simulink model "flatball_6dof_candp_wrk"  (R2021b)
settings: Solver=ode1be  StartTime=0.0  StopTime=30  FixedStep=1e-3  MaxStep=0.01  MinStep=0.01  RelTol=1e-3
values from neighbouring files (symbols this model uses):
  amb = evalin( 'base', 'amb')    [flatball_6dof_eqom.m]
  C = evalin( 'base', 'C')    [flatball_6dof_eqom.m]
  disc = evalin( 'base', 'disc')    [flatball_6dof_eqom.m]    (also in flatball_6dof_init.m = struct; flatball_init_disc_params.m = struct)
  k_launch_F_t_release = 0.60    (= 0.6)    [flatball_6dof_hucker_init.m]
  k_launch_Fx_kd = 2e-2    (= 0.02)    [flatball_6dof_hucker_init.m]
  k_launch_Fx_ki = 15    [flatball_6dof_hucker_init.m]
  k_launch_Fx_kp = 7.5    [flatball_6dof_hucker_init.m]
  k_launch_Fx_sat_hi = 150    [flatball_6dof_hucker_init.m]
  k_launch_Fx_sat_lo = -150    [flatball_6dof_hucker_init.m]
  k_launch_Fx_t_launch_begin = 0.50    (= 0.5)    [flatball_6dof_hucker_init.m]
  k_launch_Fx_t_launch_end = k_launch_F_t_release    (= 0.6)    [flatball_6dof_hucker_init.m]
  k_launch_Fy_kd = k_launch_Fx_kd    (= 0.02)    [flatball_6dof_hucker_init.m]
  k_launch_Fy_ki = k_launch_Fx_ki    (= 15)    [flatball_6dof_hucker_init.m]
  k_launch_Fy_kp = k_launch_Fx_kp    (= 7.5)    [flatball_6dof_hucker_init.m]
  k_launch_Fy_sat_hi = k_launch_Fx_sat_hi    (= 150)    [flatball_6dof_hucker_init.m]
  k_launch_Fy_sat_lo = k_launch_Fx_sat_lo    (= -150)    [flatball_6dof_hucker_init.m]
  k_launch_Fy_t_launch_begin = 0.50    (= 0.5)    [flatball_6dof_hucker_init.m]
  k_launch_Fy_t_launch_end = k_launch_F_t_release    (= 0.6)    [flatball_6dof_hucker_init.m]
  k_launch_Fz_kd = 2.5    [flatball_6dof_hucker_init.m]
  k_launch_Fz_ki = 50    [flatball_6dof_hucker_init.m]
  k_launch_Fz_kp = 20    [flatball_6dof_hucker_init.m]
  k_launch_Fz_sat_hi = 25    [flatball_6dof_hucker_init.m]
  k_launch_Fz_sat_lo = -25    [flatball_6dof_hucker_init.m]
  k_launch_Fz_t_launch_begin = 0.10    (= 0.1)    [flatball_6dof_hucker_init.m]
  k_launch_Fz_t_launch_end = k_launch_F_t_release    (= 0.6)    [flatball_6dof_hucker_init.m]
  k_launch_M_t_release = 0.60    (= 0.6)    [flatball_6dof_hucker_init.m]
  k_launch_Mx_kd = 0.125    [flatball_6dof_hucker_init.m]
  k_launch_Mx_ki = 1.125    [flatball_6dof_hucker_init.m]
  k_launch_Mx_kp = 3.5    [flatball_6dof_hucker_init.m]
  k_launch_Mx_sat_hi = 2.5    [flatball_6dof_hucker_init.m]
  k_launch_Mx_sat_lo = -2.5    [flatball_6dof_hucker_init.m]
  k_launch_Mx_t_launch_begin = 0.30    (= 0.3)    [flatball_6dof_hucker_init.m]
  k_launch_Mx_t_launch_end = k_launch_M_t_release    (= 0.6)    [flatball_6dof_hucker_init.m]
  k_launch_My_kd = 0.1125    [flatball_6dof_hucker_init.m]
  k_launch_My_ki = 5.5    [flatball_6dof_hucker_init.m]
  k_launch_My_kp = 4.25    [flatball_6dof_hucker_init.m]
  k_launch_My_sat_hi = 2.5    [flatball_6dof_hucker_init.m]
  k_launch_My_sat_lo = -2.5    [flatball_6dof_hucker_init.m]
  k_launch_My_t_launch_begin = 0.40    (= 0.4)    [flatball_6dof_hucker_init.m]
  k_launch_My_t_launch_end = k_launch_M_t_release    (= 0.6)    [flatball_6dof_hucker_init.m]
  k_launch_Mz_kd = 1e-8    (= 1e-08)    [flatball_6dof_hucker_init.m]
  k_launch_Mz_ki = 0.2575    [flatball_6dof_hucker_init.m]
  k_launch_Mz_kp = 0.25    [flatball_6dof_hucker_init.m]
  k_launch_Mz_sat_hi = 7.5    [flatball_6dof_hucker_init.m]
  k_launch_Mz_sat_lo = -7.5    [flatball_6dof_hucker_init.m]
  k_launch_Mz_t_launch_begin = 0.20    (= 0.2)    [flatball_6dof_hucker_init.m]
  k_launch_Mz_t_launch_end = k_launch_M_t_release    (= 0.6)    [flatball_6dof_hucker_init.m]
  XL_desired = [0 0 -45*C.IN2M, 5*C.DEG2RAD 5*C.DEG2RAD 0, 15 -3 0, 0 0 500*C.RPM2RADSEC]    [flatball_6dof_wrk.m]
undefined symbols (not defined in the file or in its folder): CandP, er, flatball, flatball_6dof_plnt_lib, huck, hucker_lib
libraries: slpidlib x6, simulink x5
(part 1 of 2)
settings Model: Creator=misc.protolabs@gmail.com  LastModifiedBy=schae
settings SolverCC: InitialStep=0.01  NumberNewtonIterations=10
settings DataIOCC: SaveFormat=StructureWithTime  SaveOutput=off  DSMLogging=off  SaveTime=off  ReturnWorkspaceOutputsName=simout
settings DebuggingCC: InheritedTsInSrcMsg=none

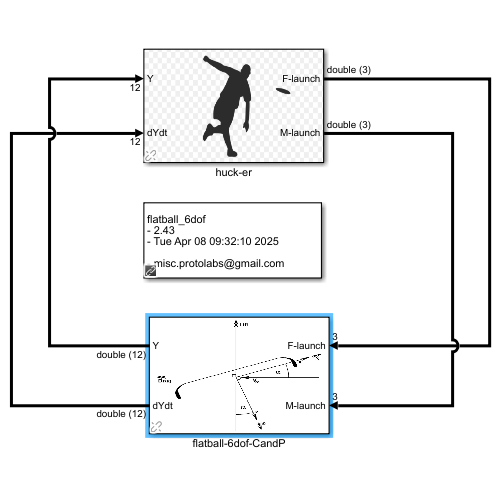
[thumbnail: Simulink's stored preview of the top-level diagram]
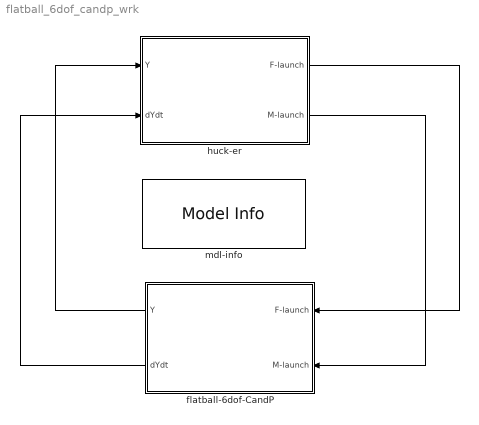
== system flatball_6dof_candp_wrk ==
  flatball-6dof-CandP : Subsystem  AncestorBlock=flatball_6dof_plnt_lib/flatball-6dof-CandP
      mask Display: image('C:\.local\desktop\flatball-dev-main-misc.protolabs\media\img\screenshots\flatball-6dof.png'); % Use "Edit Image" on toolstrip to change.
  huck-er : Subsystem  AncestorBlock=hucker_lib/huck-er
      mask Display: image('C:\.local\desktop\flatball-dev-main-misc.protolabs\media\img\screenshots\hucker.png'); % Use "Edit Image" on toolstrip to change.
  mdl-info : simulink/Model-Wide Utilities/Model Info  Frame=on  DisplayStringWithTags=|  HorizontalTextAlignment=Left  LeftAlignmentValue=0.02
      | flatball_6dof
      | - %<ModelVersion>
      | - %<LastModificationDate>
      | 
      | - %<Creator>
  wires:
  flatball-6dof-CandP/2(dYdt) -> huck-er/2(dYdt)
  flatball-6dof-CandP/1(Y) -> huck-er/1(Y)
  huck-er/1(F-launch) -> flatball-6dof-CandP/1(F-launch)
  huck-er/2(M-launch) -> flatball-6dof-CandP/2(M-launch)

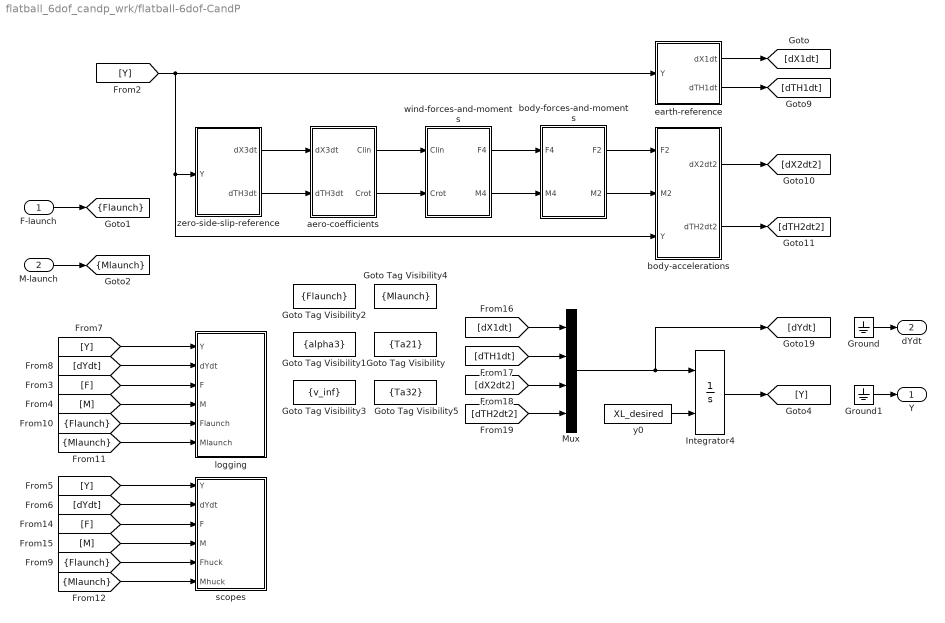
== system flatball_6dof_candp_wrk/flatball-6dof-CandP ==
  F-launch : Inport
  M-launch : Inport  Port=2
  Goto Tag Visibility : GotoTagVisibility  GotoTag=Ta21
  Goto Tag Visibility1 : GotoTagVisibility  GotoTag=alpha3
  Goto Tag Visibility2 : GotoTagVisibility  GotoTag=Flaunch
  Goto Tag Visibility3 : GotoTagVisibility  GotoTag=v_inf
  Goto Tag Visibility4 : GotoTagVisibility  GotoTag=Mlaunch
  Goto Tag Visibility5 : GotoTagVisibility  GotoTag=Ta32
  Ground : Ground
  Ground1 : Ground
  Integrator4 : Integrator  InitialConditionSource=external
  Mux : Mux
  aero-coefficients : Subsystem
  body-accelerations : Subsystem
  body-forces-and-moments : Subsystem
  earth-reference : Subsystem
  logging : Subsystem
  scopes : Subsystem
  wind-forces-and-moments : Subsystem
  y0 : Constant  Value=XL_desired
  zero-side-slip-reference : Subsystem
  Y : Outport
  dYdt : Outport  Port=2
  tag scope: Flaunch=scoped, Mlaunch=scoped
  wires:
  Ground1/1 -> Y/1
  M-launch/1 -> [Mlaunch]
  Ground/1 -> dYdt/1
  wind-forces-and-moments/2(M4) -> body-forces-and-moments/2(M4)
  body-forces-and-moments/2(M2) -> body-accelerations/2(M2)
  wind-forces-and-moments/1(F4) -> body-forces-and-moments/1(F4)
  Mux/1 -> Integrator4/1, [dYdt]
  [dX1dt] -> Mux/1
  aero-coefficients/1(Clin) -> wind-forces-and-moments/1(Clin)
  body-accelerations/1(dX2dt2) -> [dX2dt2]
  [dX2dt2] -> Mux/3
  aero-coefficients/2(Crot) -> wind-forces-and-moments/2(Crot)
  [dTH1dt] -> Mux/2
  body-forces-and-moments/1(F2) -> body-accelerations/1(F2)
  zero-side-slip-reference/2(dTH3dt) -> aero-coefficients/2(dTH3dt)
  earth-reference/1(dX1dt) -> [dX1dt]
  earth-reference/2(dTH1dt) -> [dTH1dt]
  body-accelerations/2(dTH2dt2) -> [dTH2dt2]
  [dTH2dt2] -> Mux/4
  F-launch/1 -> [Flaunch]
  Integrator4/1 -> [Y]
  zero-side-slip-reference/1(dX3dt) -> aero-coefficients/1(dX3dt)
  [Y] -> earth-reference/1(Y), body-accelerations/3(Y), zero-side-slip-reference/1(Y)
  y0/1 -> Integrator4/2
  [M] -> scopes/4(M)
  [Flaunch] -> scopes/5(Fhuck)
  [Y] -> logging/1(Y)
  [F] -> scopes/3(F)
  [Mlaunch] -> scopes/6(Mhuck)
  [M] -> logging/4(M)
  [Y] -> scopes/1(Y)
  [dYdt] -> scopes/2(dYdt)
  [Flaunch] -> logging/5(Flaunch)
  [F] -> logging/3(F)
  [Mlaunch] -> logging/6(Mlaunch)
  [dYdt] -> logging/2(dYdt)

== system flatball_6dof_candp_wrk/huck-er ==
  Y : Inport
  dYdt : Inport  Port=2
  Flaunch-ctrl : Subsystem
  Mlaunch-ctrl : Subsystem
  F-launch : Outport
  M-launch : Outport  Port=2
  wires:
  Flaunch-ctrl/1(Flaunch) -> F-launch/1
  dYdt/1 -> Flaunch-ctrl/2(dYdt), Mlaunch-ctrl/2(dYdt)
  Y/1 -> Mlaunch-ctrl/1(Y), Flaunch-ctrl/1(Y)
  Mlaunch-ctrl/1(Mlaunch) -> M-launch/1

== system flatball_6dof_candp_wrk/flatball-6dof-CandP/aero-coefficients ==
  dX3dt : Inport
  dTH3dt : Inport  Port=2
  Mux1 : Mux  Inputs=3
  Mux2 : Mux  Inputs=3
  Subsystem : Subsystem
  Subsystem1 : Subsystem
  Subsystem2 : Subsystem
  Subsystem3 : Subsystem
  Subsystem4 : Subsystem
  Subsystem5 : Subsystem
  alpha3 : Subsystem
  Clin : Outport
  Crot : Outport  Port=2
  wires:
  dX3dt/1 -> alpha3/1(dX3dt)
  Mux2/1 -> Clin/1
  dTH3dt/1 -> Subsystem3/1(dTH3dt), Subsystem2/1(dTH3dt), Subsystem4/1(dTH3dt), Subsystem5/1(dTH3dt)
  Mux1/1 -> Crot/1
  alpha3/1(alpha3) -> [alpha3]
  [alpha3] -> Subsystem/1(alpha3), Subsystem2/2(alpha3), Subsystem1/1(alpha3)
  Subsystem5/1(Cside) -> Mux2/2  "Cside"
  Subsystem/1(Cdrag) -> Mux2/1  "Cdrag"
  Subsystem1/1(Clift) -> Mux2/3  "Clift"
  Subsystem2/1(CM) -> Mux1/2  "CM"
  [v_inf] -> Subsystem5/2(v_inf), Subsystem3/2(v_inf), Subsystem2/3(v_inf), Subsystem4/2(v_inf)
  Subsystem3/1(CL) -> Mux1/1  "CL"
  Subsystem4/1(CN) -> Mux1/3  "CN"

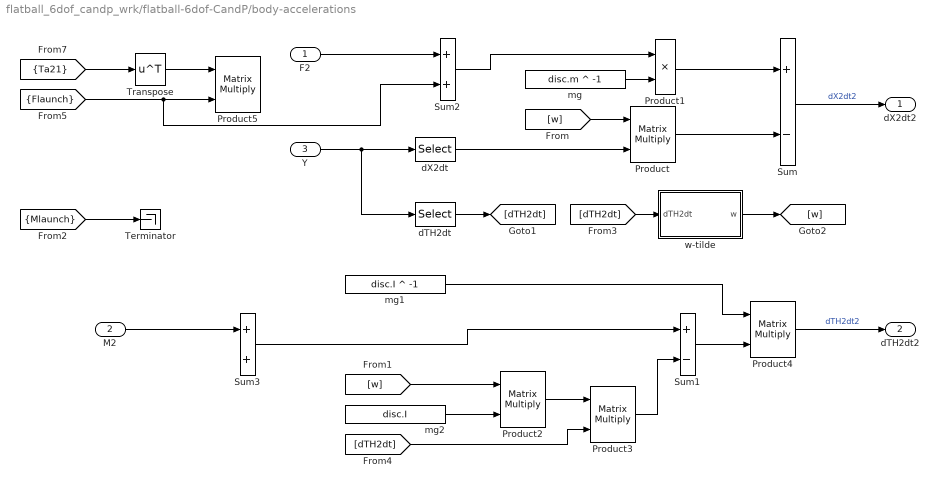
== system flatball_6dof_candp_wrk/flatball-6dof-CandP/body-accelerations ==
  F2 : Inport
  M2 : Inport  Port=2
  Y : Inport  Port=3
  Product{,2..5} (5 alike) : Product  Multiplication=Matrix(*)
  Product1 : Product  Inputs=**
  Sum : Sum  Inputs=+-
  Sum1 : Sum  Inputs=+-
  Sum2 : Sum
  Sum3 : Sum
  Terminator : Terminator
  Transpose : Math  Operator=transpose  SaturateOnIntegerOverflow=on
  dTH2dt : Selector  InputPortWidth=12  IndexOptions=Index vector (dialog)  Indices=[10 11 12]  OutputSizes=1
  dX2dt : Selector  InputPortWidth=12  IndexOptions=Index vector (dialog)  Indices=[7 8 9]  OutputSizes=1
  mg : Constant  Value=disc.m ^ -1
  mg1 : Constant  Value=disc.I ^ -1
  mg2 : Constant  Value=disc.I
  w-tilde : MATLAB Function  TreatAsAtomicUnit=on
  dX2dt2 : Outport
  dTH2dt2 : Outport  Port=2
  wires:
  Y/1 -> dTH2dt/1, dX2dt/1
  Sum/1 -> dX2dt2/1  "dX2dt2"
  Product4/1 -> dTH2dt2/1  "dTH2dt2"
  dX2dt/1 -> Product/2
  F2/1 -> Sum2/1
  mg/1 -> Product1/2
  Product1/1 -> Sum/1
  Product/1 -> Sum/2
  w-tilde/1(w) -> [w]
  [w] -> Product/1
  mg2/1 -> Product2/2
  Product2/1 -> Product3/1
  dTH2dt/1 -> [dTH2dt]
  [dTH2dt] -> w-tilde/1(dTH2dt)
  [dTH2dt] -> Product3/2
  mg1/1 -> Product4/1
  [w] -> Product2/1
  Product3/1 -> Sum1/2
  Sum1/1 -> Product4/2
  [Ta21] -> Transpose/1
  [Flaunch] -> Sum2/2, Product5/2
  Sum2/1 -> Product1/1
  Transpose/1 -> Product5/1
  [Mlaunch] -> Terminator/1
  M2/1 -> Sum3/1
  Sum3/1 -> Sum1/1

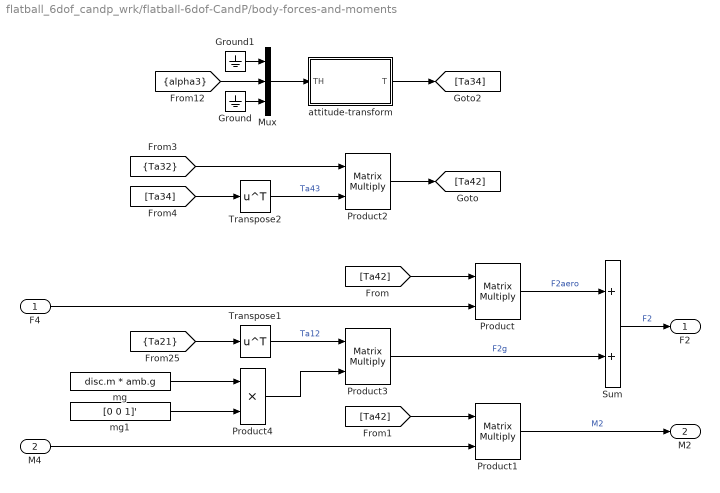
== system flatball_6dof_candp_wrk/flatball-6dof-CandP/body-forces-and-moments ==
  F4 : Inport
  M4 : Inport  Port=2
  Ground : Ground
  Ground1 : Ground
  Mux : Mux  Inputs=3
  Product{,1..3} (4 alike) : Product  Multiplication=Matrix(*)
  Product4 : Product
  Sum : Sum  Inputs=2
  Transpose1 : Math  Operator=transpose  SaturateOnIntegerOverflow=on
  Transpose2 : Math  Operator=transpose  SaturateOnIntegerOverflow=on
  attitude-transform : MATLAB Function  TreatAsAtomicUnit=on
  mg : Constant  Value=disc.m * amb.g
  mg1 : Constant  Value=[0 0 1]'
  F2 : Outport
  M2 : Outport  Port=2
  wires:
  [alpha3] -> Mux/2
  F4/1 -> Product/2
  Product/1 -> Sum/1  "F2aero"
  [Ta21] -> Transpose1/1
  Product1/1 -> M2/1  "M2"
  Ground1/1 -> Mux/1
  Mux/1 -> attitude-transform/1(TH)
  Ground/1 -> Mux/3
  attitude-transform/1(T) -> [Ta34]
  [Ta32] -> Product2/1
  [Ta34] -> Transpose2/1
  Product2/1 -> [Ta42]
  [Ta42] -> Product/1
  [Ta42] -> Product1/1
  Sum/1 -> F2/1  "F2"
  Product3/1 -> Sum/2  "F2g"
  Product4/1 -> Product3/2
  Transpose2/1 -> Product2/2  "Ta43"
  mg/1 -> Product4/1
  mg1/1 -> Product4/2
  Transpose1/1 -> Product3/1  "Ta12"
  M4/1 -> Product1/2

== system flatball_6dof_candp_wrk/flatball-6dof-CandP/earth-reference ==
  Y : Inport
  Product : Product  Multiplication=Matrix(*)
  Product1 : Product  Multiplication=Matrix(*)
  TH1 : Selector  InputPortWidth=12  IndexOptions=Index vector (dialog)  Indices=[4 5 6]  OutputSizes=1
  Terminator : Terminator
  X1 : Selector  InputPortWidth=12  IndexOptions=Index vector (dialog)  Indices=[1 2 3]  OutputSizes=1
  attitude-transform : MATLAB Function  TreatAsAtomicUnit=on
  dTH2dt : Selector  InputPortWidth=12  IndexOptions=Index vector (dialog)  Indices=[10 11 12]  OutputSizes=1
  dX2dt : Selector  InputPortWidth=12  IndexOptions=Index vector (dialog)  Indices=[7 8 9]  OutputSizes=1
  rate-transform : MATLAB Function  TreatAsAtomicUnit=on
  v_inf : Subsystem
  dX1dt : Outport
  dTH1dt : Outport  Port=2
  tag scope: Ta21=scoped
  wires:
  Y/1 -> X1/1, dTH2dt/1, dX2dt/1, TH1/1
  dX2dt/1 -> v_inf/1(dX2dt), Product/2
  TH1/1 -> rate-transform/1(TH), attitude-transform/1(TH)  "TH1"
  Product/1 -> dX1dt/1  "X1dot"
  Product1/1 -> dTH1dt/1  "TH1dot"
  X1/1 -> Terminator/1  "X1"
  attitude-transform/1(T) -> [Ta21]
  rate-transform/1(T) -> [Tr21]
  [Ta21] -> Product/1
  [Tr21] -> Product1/1
  dTH2dt/1 -> Product1/2

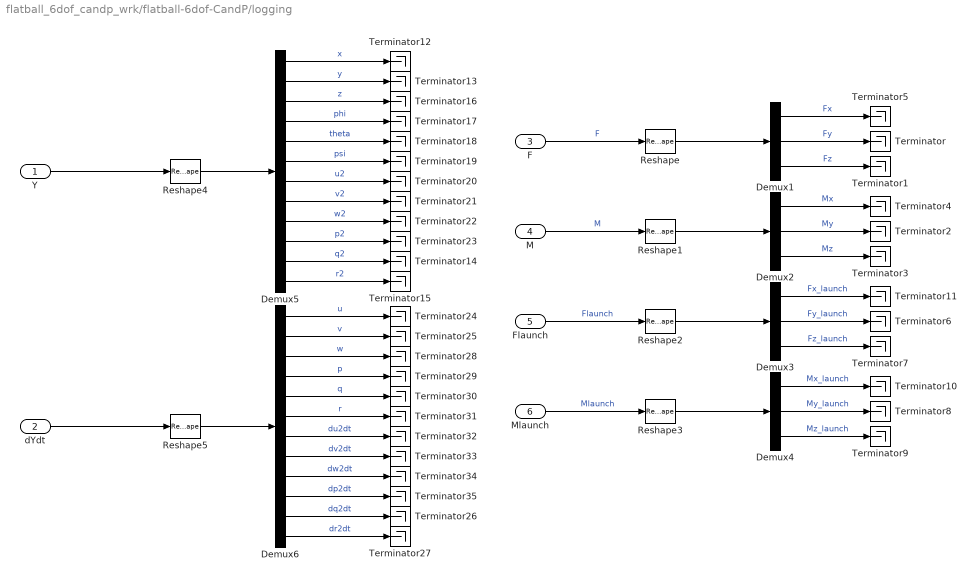
== system flatball_6dof_candp_wrk/flatball-6dof-CandP/logging ==
  Y : Inport
  dYdt : Inport  Port=2
  F : Inport  Port=3
  M : Inport  Port=4
  Flaunch : Inport  Port=5
  Mlaunch : Inport  Port=6
  Demux{1..4} (4 alike) : Demux  Outputs=3
  Demux5 : Demux  Outputs=[1 1 1 1 1 1 1 1 1 1 1 1]
  Demux6 : Demux  Outputs=[1 1 1 1 1 1 1 1 1 1 1 1]
  Reshape{,1..5} (6 alike) : Reshape
  Terminator{,1..35} (36 alike) : Terminator
  wires:
  Demux6/3 -> Terminator28/1  "w"
  Demux6/1 -> Terminator24/1  "u"
  Demux6/8 -> Terminator33/1  "dv2dt"
  Demux6/9 -> Terminator34/1  "dw2dt"
  Reshape5/1 -> Demux6/1
  Demux6/2 -> Terminator25/1  "v"
  Demux6/12 -> Terminator27/1  "dr2dt"
  Demux6/10 -> Terminator35/1  "dp2dt"
  Demux6/7 -> Terminator32/1  "du2dt"
  Demux6/5 -> Terminator30/1  "q"
  Demux6/6 -> Terminator31/1  "r"
  Demux6/11 -> Terminator26/1  "dq2dt"
  Demux6/4 -> Terminator29/1  "p"
  dYdt/1 -> Reshape5/1
  Y/1 -> Reshape4/1
  Demux5/4 -> Terminator17/1  "phi"
  Demux5/11 -> Terminator14/1  "q2"
  Demux5/6 -> Terminator19/1  "psi"
  Demux5/5 -> Terminator18/1  "theta"
  Demux5/7 -> Terminator20/1  "u2"
  Demux5/10 -> Terminator23/1  "p2"
  Demux5/12 -> Terminator15/1  "r2"
  Demux5/2 -> Terminator13/1  "y"
  Reshape4/1 -> Demux5/1
  Demux5/9 -> Terminator22/1  "w2"
  Demux5/8 -> Terminator21/1  "v2"
  Demux5/1 -> Terminator12/1  "x"
  Demux5/3 -> Terminator16/1  "z"
  Mlaunch/1 -> Reshape3/1  "Mlaunch"
  F/1 -> Reshape/1  "F"
  Demux3/2 -> Terminator6/1  "Fy_launch"
  Demux3/1 -> Terminator11/1  "Fx_launch"
  Flaunch/1 -> Reshape2/1  "Flaunch"
  Reshape3/1 -> Demux4/1
  Demux4/3 -> Terminator9/1  "Mz_launch"
  Demux4/1 -> Terminator10/1  "Mx_launch"
  Reshape/1 -> Demux1/1
  Demux1/1 -> Terminator5/1  "Fx"
  Demux4/2 -> Terminator8/1  "My_launch"
  M/1 -> Reshape1/1  "M"
  Demux3/3 -> Terminator7/1  "Fz_launch"
  Demux2/2 -> Terminator2/1  "My"
  Demux1/2 -> Terminator/1  "Fy"
  Demux1/3 -> Terminator1/1  "Fz"
  Reshape2/1 -> Demux3/1
  Demux2/1 -> Terminator4/1  "Mx"
  Demux2/3 -> Terminator3/1  "Mz"
  Reshape1/1 -> Demux2/1

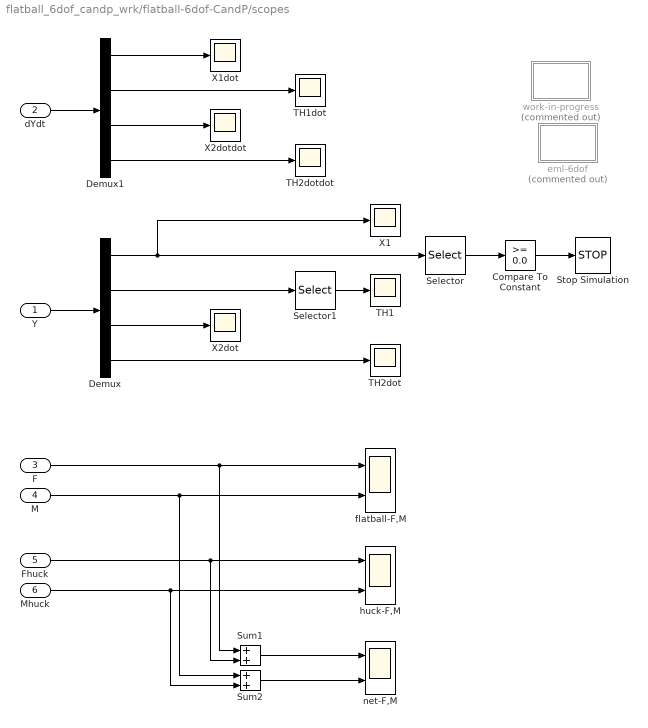
== system flatball_6dof_candp_wrk/flatball-6dof-CandP/scopes ==
  Y : Inport
  dYdt : Inport  Port=2
  F : Inport  Port=3
  M : Inport  Port=4
  Fhuck : Inport  Port=5
  Mhuck : Inport  Port=6
  Compare To Constant : simulink/Logic and Bit Operations/Compare To Constant  relop=>=  const=0.0  OutDataTypeStr=boolean
  Demux : Demux  Outputs=[3 3 3 3]
  Demux1 : Demux  Outputs=[3 3 3 3]
  Selector : Selector  InputPortWidth=3  IndexOptions=Index vector (dialog)  Indices=[3]  OutputSizes=1
  Selector1 : Selector  InputPortWidth=3  IndexOptions=Index vector (dialog)  Indices=[1 2]  OutputSizes=1
  Stop Simulation : Stop
  Sum1 : Sum
  Sum2 : Sum
  TH1 : Scope
  TH1dot : Scope
  TH2dot : Scope
  TH2dotdot : Scope
  X1 : Scope
  X1dot : Scope
  X2dot : Scope
  X2dotdot : Scope
  eml-6dof : Subsystem  Commented=on
  flatball-F,M : Scope  NumInputPorts=2
  huck-F,M : Scope  NumInputPorts=2
  net-F,M : Scope  NumInputPorts=2
  work-in-progress : Subsystem  Commented=on
  wires:
  Demux/1 -> Selector/1, X1/1
  Demux1/3 -> X2dotdot/1
  Y/1 -> Demux/1
  Compare To Constant/1 -> Stop Simulation/1
  Demux1/4 -> TH2dotdot/1
  Demux/3 -> X2dot/1
  Demux1/1 -> X1dot/1
  Selector1/1 -> TH1/1
  Demux/2 -> Selector1/1
  Demux1/2 -> TH1dot/1
  Selector/1 -> Compare To Constant/1
  dYdt/1 -> Demux1/1
  Demux/4 -> TH2dot/1
  M/1 -> flatball-F,M/2, Sum2/1
  F/1 -> flatball-F,M/1, Sum1/1
  Fhuck/1 -> huck-F,M/1, Sum1/2
  Sum1/1 -> net-F,M/1
  Mhuck/1 -> huck-F,M/2, Sum2/2
  Sum2/1 -> net-F,M/2

== system flatball_6dof_candp_wrk/flatball-6dof-CandP/wind-forces-and-moments ==
  Clin : Inport
  Crot : Inport  Port=2
  Demux : Demux  Outputs=3
  Demux1 : Demux  Outputs=3
  Gain{,1..3} (4 alike) : Gain  Gain=-1
  Gain4 : Gain  Gain=0
  Mux : Mux  Inputs=3
  Product : Product
  Product1 : Product
  Subsystem : Subsystem
  Terminator : Terminator
  Terminator1 : Terminator
  Terminator2 : Terminator
  F4 : Outport
  M4 : Outport  Port=2
  wires:
  Product/1 -> [F4], F4/1  "F4"
  Product1/1 -> M4/1  "M4"
  Demux/2 -> Terminator1/1
  Demux/1 -> Gain/1
  Demux/3 -> Gain1/1
  [F4] -> Demux/1
  Gain1/1 -> Terminator2/1  "lift"
  Gain/1 -> Terminator/1  "drag"
  Demux1/3 -> Gain3/1
  Clin/1 -> Demux1/1
  Demux1/2 -> Gain4/1
  Demux1/1 -> Gain2/1
  Gain3/1 -> Mux/3
  Gain4/1 -> Mux/2
  Gain2/1 -> Mux/1
  Mux/1 -> Product/1
  Subsystem/1(qS) -> Product/2
  Subsystem/2(qSc) -> Product1/1
  Crot/1 -> Product1/2
  [v_inf] -> Subsystem/1(v_inf)

== system flatball_6dof_candp_wrk/flatball-6dof-CandP/zero-side-slip-reference ==
  Y : Inport
  Ground : Ground
  Ground1 : Ground
  Mux : Mux  Inputs=3
  Product : Product  Multiplication=Matrix(*)
  Product1 : Product  Multiplication=Matrix(*)
  Transpose : Math  Operator=transpose  SaturateOnIntegerOverflow=on
  attitude-transform : MATLAB Function  TreatAsAtomicUnit=on
  beta2 : Subsystem
  dTH2dt : Selector  InputPortWidth=12  IndexOptions=Index vector (dialog)  Indices=[10 11 12]  OutputSizes=1
  dX2dt : Selector  InputPortWidth=12  IndexOptions=Index vector (dialog)  Indices=[7 8 9]  OutputSizes=1
  dX3dt : Outport
  dTH3dt : Outport  Port=2
  tag scope: Ta32=scoped
  wires:
  Y/1 -> dX2dt/1, dTH2dt/1
  Product1/1 -> dTH3dt/1  "dTH3dt"
  Product/1 -> dX3dt/1  "dX3dt"
  dX2dt/1 -> beta2/1(dX2dt), Product/2  "dX2dt"
  dTH2dt/1 -> Product1/2  "dTH2dt"
  beta2/1(beta2) -> Mux/3
  Mux/1 -> attitude-transform/1(TH)
  Ground/1 -> Mux/2
  Ground1/1 -> Mux/1
  attitude-transform/1(T) -> [Ta32]
  [Ta23] -> Product1/1, Product/1
  [Ta32] -> Transpose/1
  Transpose/1 -> [Ta23]  "Ta23"

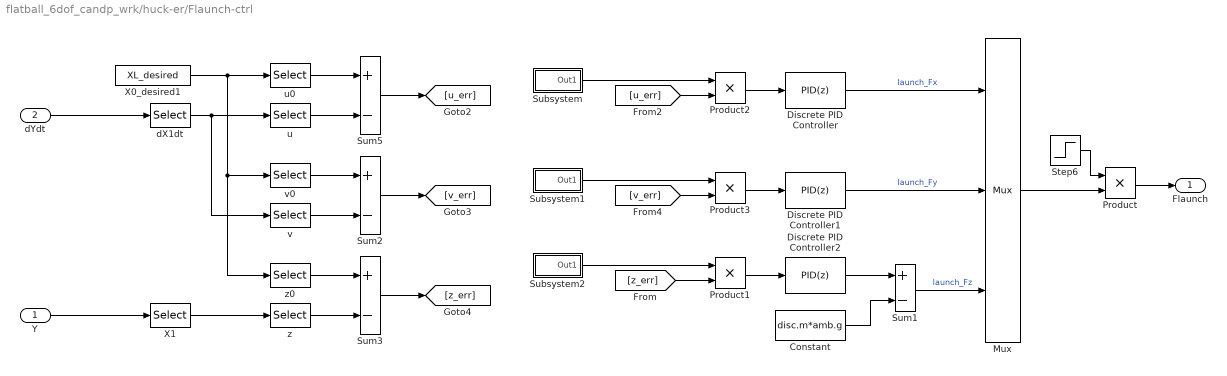
== system flatball_6dof_candp_wrk/huck-er/Flaunch-ctrl ==
  Y : Inport
  dYdt : Inport  Port=2
  Constant : Constant  Value=disc.m*amb.g
  Discrete PID Controller : slpidlib/PID Controller  Controller=PID  Form=Parallel  TimeDomain=Discrete-time  UseExternalTs=off  SampleTime=-1  IntegratorMethod=Forward Euler  FilterMethod=Forward Euler  ControllerParametersSource=internal  P=k_launch_Fx_kp  I=k_launch_Fx_ki  D=k_launch_Fx_kd  UseFilter=on  N=100  TunerSelectOption=Transfer Function Based (PID Tuner App)  InitialConditionSource=internal  InitialConditionForIntegrator=0  InitialConditionForFilter=0  DifferentiatorICPrevScaledInput=0  ExternalReset=none  TrackingMode=off  Kt=1  LimitOutput=on  SatLimitsSource=internal  UpperSaturationLimit=k_launch_Fx_sat_hi  LowerSaturationLimit=k_launch_Fx_sat_lo  LinearizeAsGain=off  AntiWindupMode=clamping  Kb=1  POutMin=[]  POutMax=[]  IOutMin=[]  IOutMax=[]  DOutMin=[]  DOutMax=[]  NOutMin=[]  NOutMax=[]  SumOutMin=[]  SumOutMax=[]  SaturationOutMin=[]  SaturationOutMax=[]  PParamMin=[]  PParamMax=[]  IParamMin=[]  IParamMax=[]  DParamMin=[]  DParamMax=[]  NParamMin=[]  NParamMax=[]  KbParamMin=[]  KbParamMax=[]  KtParamMin=[]  KtParamMax=[]  KbOutMin=[]  KbOutMax=[]  KtOutMin=[]  KtOutMax=[]  IntegratorOutMin=[]  IntegratorOutMax=[]  FilterOutMin=[]  FilterOutMax=[]  SumI1OutMin=[]  SumI1OutMax=[]  SumI2OutMin=[]  SumI2OutMax=[]  SumI3OutMin=[]  SumI3OutMax=[]  SumI4OutMin=[]  SumI4OutMax=[]  SumDOutMin=[]  SumDOutMax=[]  DifferentiatorOutMin=[]  DifferentiatorOutMax=[]  FilterDiffOutCoefMin=[]  FilterDiffOutCoefMax=[]  ReciprocalOutMin=[]  ReciprocalOutMax=[]  SumDenOutMin=[]  SumDenOutMax=[]  SumNumOutMin=[]  SumNumOutMax=[]  DivideOutMin=[]  DivideOutMax=[]  UdiffTsProdOutMin=[]  UdiffTsProdOutMax=[]  NTsProdOutMin=[]  NTsProdOutMax=[]  UintegralTsProdOutMin=[]  UintegralTsProdOutMax=[]  UngainTsProdOutMin=[]  UngainTsProdOutMax=[]  IntegratorContinuousStateAttributes=''  IntegratorStateMustResolveToSignalObject=off  IntegratorRTWStateStorageClass=Auto  FilterContinuousStateAttributes=''  FilterStateMustResolveToSignalObject=off  FilterRTWStateStorageClass=Auto  ParallelPVariant=InternalParameters  IdealPVariant=Disabled  IVariant=InternalParameters  DVariant=InternalParameters  IntegratorVariant=Discrete  SatVariant=Enabled  AWVariant=DiscClampingParallel  PCopyVariant=Disabled  TRVariant=Disabled  FdbkBlocksVariant=Forward  IdealPFdbkVariant=Disabled  SatFdbkVariant=Disabled  DerivativeFilterVariant=ForwardEulerFilter  NVariant=InternalParameters  NCopyVariant=Disabled  FilterICVariant=InternalICsFilter  IntegratorICVariant=InternalICs  ExternalResetVariant=Disabled  TRSumVariant=Passthrough  SumFdbkVariant=Disabled  SumVariant=Sum_PID  TsampFilterVariant=InternalTs  TsampNgainVariant=Passthrough  TsampIntegralVariant=Passthrough  ExternalSaturationOutDataTypeStr=Inherit: Same as second input
  Discrete PID Controller1 : slpidlib/PID Controller  Controller=PID  Form=Parallel  TimeDomain=Discrete-time  UseExternalTs=off  SampleTime=-1  IntegratorMethod=Forward Euler  FilterMethod=Forward Euler  ControllerParametersSource=internal  P=k_launch_Fy_kp  I=k_launch_Fy_ki  D=k_launch_Fy_kd  UseFilter=on  N=100  TunerSelectOption=Transfer Function Based (PID Tuner App)  InitialConditionSource=internal  InitialConditionForIntegrator=0  InitialConditionForFilter=0  DifferentiatorICPrevScaledInput=0  ExternalReset=none  TrackingMode=off  Kt=1  LimitOutput=on  SatLimitsSource=internal  UpperSaturationLimit=k_launch_Fy_sat_hi  LowerSaturationLimit=k_launch_Fy_sat_lo  LinearizeAsGain=off  AntiWindupMode=clamping  Kb=1  POutMin=[]  POutMax=[]  IOutMin=[]  IOutMax=[]  DOutMin=[]  DOutMax=[]  NOutMin=[]  NOutMax=[]  SumOutMin=[]  SumOutMax=[]  SaturationOutMin=[]  SaturationOutMax=[]  PParamMin=[]  PParamMax=[]  IParamMin=[]  IParamMax=[]  DParamMin=[]  DParamMax=[]  NParamMin=[]  NParamMax=[]  KbParamMin=[]  KbParamMax=[]  KtParamMin=[]  KtParamMax=[]  KbOutMin=[]  KbOutMax=[]  KtOutMin=[]  KtOutMax=[]  IntegratorOutMin=[]  IntegratorOutMax=[]  FilterOutMin=[]  FilterOutMax=[]  SumI1OutMin=[]  SumI1OutMax=[]  SumI2OutMin=[]  SumI2OutMax=[]  SumI3OutMin=[]  SumI3OutMax=[]  SumI4OutMin=[]  SumI4OutMax=[]  SumDOutMin=[]  SumDOutMax=[]  DifferentiatorOutMin=[]  DifferentiatorOutMax=[]  FilterDiffOutCoefMin=[]  FilterDiffOutCoefMax=[]  ReciprocalOutMin=[]  ReciprocalOutMax=[]  SumDenOutMin=[]  SumDenOutMax=[]  SumNumOutMin=[]  SumNumOutMax=[]  DivideOutMin=[]  DivideOutMax=[]  UdiffTsProdOutMin=[]  UdiffTsProdOutMax=[]  NTsProdOutMin=[]  NTsProdOutMax=[]  UintegralTsProdOutMin=[]  UintegralTsProdOutMax=[]  UngainTsProdOutMin=[]  UngainTsProdOutMax=[]  IntegratorContinuousStateAttributes=''  IntegratorStateMustResolveToSignalObject=off  IntegratorRTWStateStorageClass=Auto  FilterContinuousStateAttributes=''  FilterStateMustResolveToSignalObject=off  FilterRTWStateStorageClass=Auto  ParallelPVariant=InternalParameters  IdealPVariant=Disabled  IVariant=InternalParameters  DVariant=InternalParameters  IntegratorVariant=Discrete  SatVariant=Enabled  AWVariant=DiscClampingParallel  PCopyVariant=Disabled  TRVariant=Disabled  FdbkBlocksVariant=Forward  IdealPFdbkVariant=Disabled  SatFdbkVariant=Disabled  DerivativeFilterVariant=ForwardEulerFilter  NVariant=InternalParameters  NCopyVariant=Disabled  FilterICVariant=InternalICsFilter  IntegratorICVariant=InternalICs  ExternalResetVariant=Disabled  TRSumVariant=Passthrough  SumFdbkVariant=Disabled  SumVariant=Sum_PID  TsampFilterVariant=InternalTs  TsampNgainVariant=Passthrough  TsampIntegralVariant=Passthrough  ExternalSaturationOutDataTypeStr=Inherit: Same as second input
  Discrete PID Controller2 : slpidlib/PID Controller  Controller=PID  Form=Parallel  TimeDomain=Discrete-time  UseExternalTs=off  SampleTime=-1  IntegratorMethod=Forward Euler  FilterMethod=Forward Euler  ControllerParametersSource=internal  P=k_launch_Fz_kp  I=k_launch_Fz_ki  D=k_launch_Fz_kd  UseFilter=on  N=100  TunerSelectOption=Transfer Function Based (PID Tuner App)  InitialConditionSource=internal  InitialConditionForIntegrator=0  InitialConditionForFilter=0  DifferentiatorICPrevScaledInput=0  ExternalReset=none  TrackingMode=off  Kt=1  LimitOutput=on  SatLimitsSource=internal  UpperSaturationLimit=k_launch_Fz_sat_hi  LowerSaturationLimit=k_launch_Fz_sat_lo  LinearizeAsGain=off  AntiWindupMode=clamping  Kb=1  POutMin=[]  POutMax=[]  IOutMin=[]  IOutMax=[]  DOutMin=[]  DOutMax=[]  NOutMin=[]  NOutMax=[]  SumOutMin=[]  SumOutMax=[]  SaturationOutMin=[]  SaturationOutMax=[]  PParamMin=[]  PParamMax=[]  IParamMin=[]  IParamMax=[]  DParamMin=[]  DParamMax=[]  NParamMin=[]  NParamMax=[]  KbParamMin=[]  KbParamMax=[]  KtParamMin=[]  KtParamMax=[]  KbOutMin=[]  KbOutMax=[]  KtOutMin=[]  KtOutMax=[]  IntegratorOutMin=[]  IntegratorOutMax=[]  FilterOutMin=[]  FilterOutMax=[]  SumI1OutMin=[]  SumI1OutMax=[]  SumI2OutMin=[]  SumI2OutMax=[]  SumI3OutMin=[]  SumI3OutMax=[]  SumI4OutMin=[]  SumI4OutMax=[]  SumDOutMin=[]  SumDOutMax=[]  DifferentiatorOutMin=[]  DifferentiatorOutMax=[]  FilterDiffOutCoefMin=[]  FilterDiffOutCoefMax=[]  ReciprocalOutMin=[]  ReciprocalOutMax=[]  SumDenOutMin=[]  SumDenOutMax=[]  SumNumOutMin=[]  SumNumOutMax=[]  DivideOutMin=[]  DivideOutMax=[]  UdiffTsProdOutMin=[]  UdiffTsProdOutMax=[]  NTsProdOutMin=[]  NTsProdOutMax=[]  UintegralTsProdOutMin=[]  UintegralTsProdOutMax=[]  UngainTsProdOutMin=[]  UngainTsProdOutMax=[]  IntegratorContinuousStateAttributes=''  IntegratorStateMustResolveToSignalObject=off  IntegratorRTWStateStorageClass=Auto  FilterContinuousStateAttributes=''  FilterStateMustResolveToSignalObject=off  FilterRTWStateStorageClass=Auto  ParallelPVariant=InternalParameters  IdealPVariant=Disabled  IVariant=InternalParameters  DVariant=InternalParameters  IntegratorVariant=Discrete  SatVariant=Enabled  AWVariant=DiscClampingParallel  PCopyVariant=Disabled  TRVariant=Disabled  FdbkBlocksVariant=Forward  IdealPFdbkVariant=Disabled  SatFdbkVariant=Disabled  DerivativeFilterVariant=ForwardEulerFilter  NVariant=InternalParameters  NCopyVariant=Disabled  FilterICVariant=InternalICsFilter  IntegratorICVariant=InternalICs  ExternalResetVariant=Disabled  TRSumVariant=Passthrough  SumFdbkVariant=Disabled  SumVariant=Sum_PID  TsampFilterVariant=InternalTs  TsampNgainVariant=Passthrough  TsampIntegralVariant=Passthrough  ExternalSaturationOutDataTypeStr=Inherit: Same as second input
  Mux : Mux  Inputs=3
  Product{,1..3} (4 alike) : Product
  Step6 : Step  Time=k_launch_F_t_release  Before=1  After=0
  Subsystem : Subsystem
  Subsystem1 : Subsystem
  Subsystem2 : Subsystem
  Sum{1..3,5} (4 alike) : Sum  Inputs=+-
  X0_desired1 : Constant  Value=XL_desired
  X1 : Selector  InputPortWidth=12  IndexOptions=Index vector (dialog)  Indices=[1 2 3]  OutputSizes=1
  dX1dt : Selector  InputPortWidth=12  IndexOptions=Index vector (dialog)  Indices=[1 2 3]  OutputSizes=1
  u : Selector  InputPortWidth=3  IndexOptions=Index vector (dialog)  Indices=[1]  OutputSizes=1
  u0 : Selector  InputPortWidth=12  IndexOptions=Index vector (dialog)  Indices=[7]  OutputSizes=1
  v : Selector  InputPortWidth=3  IndexOptions=Index vector (dialog)  Indices=[2]  OutputSizes=1
  v0 : Selector  InputPortWidth=12  IndexOptions=Index vector (dialog)  Indices=[8]  OutputSizes=1
  z : Selector  InputPortWidth=3  IndexOptions=Index vector (dialog)  Indices=[3]  OutputSizes=1
  z0 : Selector  InputPortWidth=12  IndexOptions=Index vector (dialog)  Indices=[3]  OutputSizes=1
  Flaunch : Outport
  wires:
  Discrete PID Controller/1 -> Mux/1  "launch_Fx"
  Discrete PID Controller1/1 -> Mux/2  "launch_Fy"
  Sum1/1 -> Mux/3  "launch_Fz"
  Step6/1 -> Product/1
  Product/1 -> Flaunch/1
  Discrete PID Controller2/1 -> Sum1/1
  Constant/1 -> Sum1/2
  Sum5/1 -> [u_err]
  dYdt/1 -> dX1dt/1
  dX1dt/1 -> v/1, u/1
  u/1 -> Sum5/2
  X0_desired1/1 -> u0/1, z0/1, v0/1
  u0/1 -> Sum5/1
  [u_err] -> Product2/2
  Y/1 -> X1/1
  Mux/1 -> Product/2
  Sum2/1 -> [v_err]
  [v_err] -> Product3/2
  v0/1 -> Sum2/1
  v/1 -> Sum2/2
  X1/1 -> z/1
  z/1 -> Sum3/2
  z0/1 -> Sum3/1
  Sum3/1 -> [z_err]
  [z_err] -> Product1/2
  Subsystem2/1(Out1) -> Product1/1
  Product2/1 -> Discrete PID Controller/1
  Product3/1 -> Discrete PID Controller1/1
  Product1/1 -> Discrete PID Controller2/1
  Subsystem1/1(Out1) -> Product3/1
  Subsystem/1(Out1) -> Product2/1

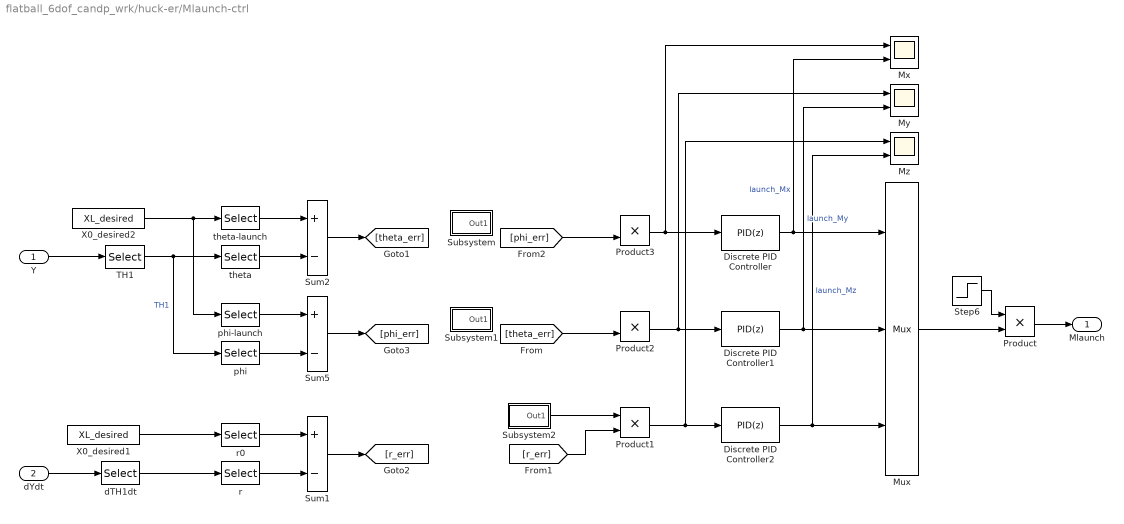
== system flatball_6dof_candp_wrk/huck-er/Mlaunch-ctrl ==
  Y : Inport
  dYdt : Inport  Port=2
  Discrete PID Controller : slpidlib/PID Controller  Controller=PID  Form=Parallel  TimeDomain=Discrete-time  UseExternalTs=off  SampleTime=-1  IntegratorMethod=Forward Euler  FilterMethod=Forward Euler  ControllerParametersSource=internal  P=k_launch_Mx_kp  I=k_launch_Mx_ki  D=k_launch_Mx_kd  UseFilter=on  N=100  TunerSelectOption=Transfer Function Based (PID Tuner App)  InitialConditionSource=internal  InitialConditionForIntegrator=0  InitialConditionForFilter=0  DifferentiatorICPrevScaledInput=0  ExternalReset=none  TrackingMode=off  Kt=1  LimitOutput=on  SatLimitsSource=internal  UpperSaturationLimit=k_launch_Mx_sat_hi  LowerSaturationLimit=k_launch_Mx_sat_lo  LinearizeAsGain=off  AntiWindupMode=clamping  Kb=1  POutMin=[]  POutMax=[]  IOutMin=[]  IOutMax=[]  DOutMin=[]  DOutMax=[]  NOutMin=[]  NOutMax=[]  SumOutMin=[]  SumOutMax=[]  SaturationOutMin=[]  SaturationOutMax=[]  PParamMin=[]  PParamMax=[]  IParamMin=[]  IParamMax=[]  DParamMin=[]  DParamMax=[]  NParamMin=[]  NParamMax=[]  KbParamMin=[]  KbParamMax=[]  KtParamMin=[]  KtParamMax=[]  KbOutMin=[]  KbOutMax=[]  KtOutMin=[]  KtOutMax=[]  IntegratorOutMin=[]  IntegratorOutMax=[]  FilterOutMin=[]  FilterOutMax=[]  SumI1OutMin=[]  SumI1OutMax=[]  SumI2OutMin=[]  SumI2OutMax=[]  SumI3OutMin=[]  SumI3OutMax=[]  SumI4OutMin=[]  SumI4OutMax=[]  SumDOutMin=[]  SumDOutMax=[]  DifferentiatorOutMin=[]  DifferentiatorOutMax=[]  FilterDiffOutCoefMin=[]  FilterDiffOutCoefMax=[]  ReciprocalOutMin=[]  ReciprocalOutMax=[]  SumDenOutMin=[]  SumDenOutMax=[]  SumNumOutMin=[]  SumNumOutMax=[]  DivideOutMin=[]  DivideOutMax=[]  UdiffTsProdOutMin=[]  UdiffTsProdOutMax=[]  NTsProdOutMin=[]  NTsProdOutMax=[]  UintegralTsProdOutMin=[]  UintegralTsProdOutMax=[]  UngainTsProdOutMin=[]  UngainTsProdOutMax=[]  IntegratorContinuousStateAttributes=''  IntegratorStateMustResolveToSignalObject=off  IntegratorRTWStateStorageClass=Auto  FilterContinuousStateAttributes=''  FilterStateMustResolveToSignalObject=off  FilterRTWStateStorageClass=Auto  ParallelPVariant=InternalParameters  IdealPVariant=Disabled  IVariant=InternalParameters  DVariant=InternalParameters  IntegratorVariant=Discrete  SatVariant=Enabled  AWVariant=DiscClampingParallel  PCopyVariant=Disabled  TRVariant=Disabled  FdbkBlocksVariant=Forward  IdealPFdbkVariant=Disabled  SatFdbkVariant=Disabled  DerivativeFilterVariant=ForwardEulerFilter  NVariant=InternalParameters  NCopyVariant=Disabled  FilterICVariant=InternalICsFilter  IntegratorICVariant=InternalICs  ExternalResetVariant=Disabled  TRSumVariant=Passthrough  SumFdbkVariant=Disabled  SumVariant=Sum_PID  TsampFilterVariant=InternalTs  TsampNgainVariant=Passthrough  TsampIntegralVariant=Passthrough  ExternalSaturationOutDataTypeStr=Inherit: Same as second input
  Discrete PID Controller1 : slpidlib/PID Controller  Controller=PID  Form=Parallel  TimeDomain=Discrete-time  UseExternalTs=off  SampleTime=-1  IntegratorMethod=Forward Euler  FilterMethod=Forward Euler  ControllerParametersSource=internal  P=k_launch_My_kp  I=k_launch_My_ki  D=k_launch_My_kd  UseFilter=on  N=100  TunerSelectOption=Transfer Function Based (PID Tuner App)  InitialConditionSource=internal  InitialConditionForIntegrator=0  InitialConditionForFilter=0  DifferentiatorICPrevScaledInput=0  ExternalReset=none  TrackingMode=off  Kt=1  LimitOutput=on  SatLimitsSource=internal  UpperSaturationLimit=k_launch_My_sat_hi  LowerSaturationLimit=k_launch_My_sat_lo  LinearizeAsGain=off  AntiWindupMode=clamping  Kb=1  POutMin=[]  POutMax=[]  IOutMin=[]  IOutMax=[]  DOutMin=[]  DOutMax=[]  NOutMin=[]  NOutMax=[]  SumOutMin=[]  SumOutMax=[]  SaturationOutMin=[]  SaturationOutMax=[]  PParamMin=[]  PParamMax=[]  IParamMin=[]  IParamMax=[]  DParamMin=[]  DParamMax=[]  NParamMin=[]  NParamMax=[]  KbParamMin=[]  KbParamMax=[]  KtParamMin=[]  KtParamMax=[]  KbOutMin=[]  KbOutMax=[]  KtOutMin=[]  KtOutMax=[]  IntegratorOutMin=[]  IntegratorOutMax=[]  FilterOutMin=[]  FilterOutMax=[]  SumI1OutMin=[]  SumI1OutMax=[]  SumI2OutMin=[]  SumI2OutMax=[]  SumI3OutMin=[]  SumI3OutMax=[]  SumI4OutMin=[]  SumI4OutMax=[]  SumDOutMin=[]  SumDOutMax=[]  DifferentiatorOutMin=[]  DifferentiatorOutMax=[]  FilterDiffOutCoefMin=[]  FilterDiffOutCoefMax=[]  ReciprocalOutMin=[]  ReciprocalOutMax=[]  SumDenOutMin=[]  SumDenOutMax=[]  SumNumOutMin=[]  SumNumOutMax=[]  DivideOutMin=[]  DivideOutMax=[]  UdiffTsProdOutMin=[]  UdiffTsProdOutMax=[]  NTsProdOutMin=[]  NTsProdOutMax=[]  UintegralTsProdOutMin=[]  UintegralTsProdOutMax=[]  UngainTsProdOutMin=[]  UngainTsProdOutMax=[]  IntegratorContinuousStateAttributes=''  IntegratorStateMustResolveToSignalObject=off  IntegratorRTWStateStorageClass=Auto  FilterContinuousStateAttributes=''  FilterStateMustResolveToSignalObject=off  FilterRTWStateStorageClass=Auto  ParallelPVariant=InternalParameters  IdealPVariant=Disabled  IVariant=InternalParameters  DVariant=InternalParameters  IntegratorVariant=Discrete  SatVariant=Enabled  AWVariant=DiscClampingParallel  PCopyVariant=Disabled  TRVariant=Disabled  FdbkBlocksVariant=Forward  IdealPFdbkVariant=Disabled  SatFdbkVariant=Disabled  DerivativeFilterVariant=ForwardEulerFilter  NVariant=InternalParameters  NCopyVariant=Disabled  FilterICVariant=InternalICsFilter  IntegratorICVariant=InternalICs  ExternalResetVariant=Disabled  TRSumVariant=Passthrough  SumFdbkVariant=Disabled  SumVariant=Sum_PID  TsampFilterVariant=InternalTs  TsampNgainVariant=Passthrough  TsampIntegralVariant=Passthrough  ExternalSaturationOutDataTypeStr=Inherit: Same as second input
  Discrete PID Controller2 : slpidlib/PID Controller  Controller=PID  Form=Parallel  TimeDomain=Discrete-time  UseExternalTs=off  SampleTime=-1  IntegratorMethod=Forward Euler  FilterMethod=Forward Euler  ControllerParametersSource=internal  P=k_launch_Mz_kp  I=k_launch_Mz_ki  D=k_launch_Mz_kd  UseFilter=on  N=100  TunerSelectOption=Transfer Function Based (PID Tuner App)  InitialConditionSource=internal  InitialConditionForIntegrator=0  InitialConditionForFilter=0  DifferentiatorICPrevScaledInput=0  ExternalReset=none  TrackingMode=off  Kt=1  LimitOutput=on  SatLimitsSource=internal  UpperSaturationLimit=k_launch_Mz_sat_hi  LowerSaturationLimit=k_launch_Mz_sat_lo  LinearizeAsGain=off  AntiWindupMode=none  Kb=1  POutMin=[]  POutMax=[]  IOutMin=[]  IOutMax=[]  DOutMin=[]  DOutMax=[]  NOutMin=[]  NOutMax=[]  SumOutMin=[]  SumOutMax=[]  SaturationOutMin=[]  SaturationOutMax=[]  PParamMin=[]  PParamMax=[]  IParamMin=[]  IParamMax=[]  DParamMin=[]  DParamMax=[]  NParamMin=[]  NParamMax=[]  KbParamMin=[]  KbParamMax=[]  KtParamMin=[]  KtParamMax=[]  KbOutMin=[]  KbOutMax=[]  KtOutMin=[]  KtOutMax=[]  IntegratorOutMin=[]  IntegratorOutMax=[]  FilterOutMin=[]  FilterOutMax=[]  SumI1OutMin=[]  SumI1OutMax=[]  SumI2OutMin=[]  SumI2OutMax=[]  SumI3OutMin=[]  SumI3OutMax=[]  SumI4OutMin=[]  SumI4OutMax=[]  SumDOutMin=[]  SumDOutMax=[]  DifferentiatorOutMin=[]  DifferentiatorOutMax=[]  FilterDiffOutCoefMin=[]  FilterDiffOutCoefMax=[]  ReciprocalOutMin=[]  ReciprocalOutMax=[]  SumDenOutMin=[]  SumDenOutMax=[]  SumNumOutMin=[]  SumNumOutMax=[]  DivideOutMin=[]  DivideOutMax=[]  UdiffTsProdOutMin=[]  UdiffTsProdOutMax=[]  NTsProdOutMin=[]  NTsProdOutMax=[]  UintegralTsProdOutMin=[]  UintegralTsProdOutMax=[]  UngainTsProdOutMin=[]  UngainTsProdOutMax=[]  IntegratorContinuousStateAttributes=''  IntegratorStateMustResolveToSignalObject=off  IntegratorRTWStateStorageClass=Auto  FilterContinuousStateAttributes=''  FilterStateMustResolveToSignalObject=off  FilterRTWStateStorageClass=Auto  ParallelPVariant=InternalParameters  IdealPVariant=Disabled  IVariant=InternalParameters  DVariant=InternalParameters  IntegratorVariant=Discrete  SatVariant=Enabled  AWVariant=Passthrough  PCopyVariant=Disabled  TRVariant=Disabled  FdbkBlocksVariant=Forward  IdealPFdbkVariant=Disabled  SatFdbkVariant=Disabled  DerivativeFilterVariant=ForwardEulerFilter  NVariant=InternalParameters  NCopyVariant=Disabled  FilterICVariant=InternalICsFilter  IntegratorICVariant=InternalICs  ExternalResetVariant=Disabled  TRSumVariant=Passthrough  SumFdbkVariant=Disabled  SumVariant=Sum_PID  TsampFilterVariant=InternalTs  TsampNgainVariant=Passthrough  TsampIntegralVariant=Passthrough  ExternalSaturationOutDataTypeStr=Inherit: Same as second input
  Mux : Mux  Inputs=3
  Mx : Scope  NumInputPorts=2
  My : Scope  NumInputPorts=2
  Mz : Scope  NumInputPorts=2
  Product{,1..3} (4 alike) : Product
  Step6 : Step  Time=k_launch_M_t_release  Before=1  After=0
  Subsystem : Subsystem
  Subsystem1 : Subsystem
  Subsystem2 : Subsystem
  Sum1 : Sum  Inputs=+-
  Sum2 : Sum  Inputs=+-
  Sum5 : Sum  Inputs=+-
  TH1 : Selector  InputPortWidth=12  IndexOptions=Index vector (dialog)  Indices=[4 5 6]  OutputSizes=1
  X0_desired1 : Constant  Value=XL_desired
  X0_desired2 : Constant  Value=XL_desired
  dTH1dt : Selector  InputPortWidth=12  IndexOptions=Index vector (dialog)  Indices=[4 5 6]  OutputSizes=1
  phi : Selector  InputPortWidth=3  IndexOptions=Index vector (dialog)  Indices=[1]  OutputSizes=1
  phi-launch : Selector  InputPortWidth=12  IndexOptions=Index vector (dialog)  Indices=[4]  OutputSizes=1
  r : Selector  InputPortWidth=3  IndexOptions=Index vector (dialog)  Indices=[3]  OutputSizes=1
  r0 : Selector  InputPortWidth=12  IndexOptions=Index vector (dialog)  Indices=[12]  OutputSizes=1
  theta : Selector  InputPortWidth=3  IndexOptions=Index vector (dialog)  Indices=[2]  OutputSizes=1
  "theta-launch " : Selector  InputPortWidth=12  IndexOptions=Index vector (dialog)  Indices=[5]  OutputSizes=1
  Mlaunch : Outport
  wires:
  Discrete PID Controller/1 -> Mux/1, Mx/2  "launch_Mx"
  Discrete PID Controller2/1 -> Mux/3, Mz/2  "launch_Mz"
  Mux/1 -> Product/2
  Step6/1 -> Product/1
  Product/1 -> Mlaunch/1
  Discrete PID Controller1/1 -> Mux/2, My/2  "launch_My"
  Product1/1 -> Discrete PID Controller2/1, Mz/1
  Product2/1 -> Discrete PID Controller1/1, My/1
  Product3/1 -> Discrete PID Controller/1, Mx/1
  Y/1 -> TH1/1
  TH1/1 -> phi/1, theta/1  "TH1"
  Subsystem2/1(Out1) -> Product1/1
  r0/1 -> Sum1/1
  dTH1dt/1 -> r/1
  r/1 -> Sum1/2
  X0_desired1/1 -> r0/1
  Sum1/1 -> [r_err]
  dYdt/1 -> dTH1dt/1
  [r_err] -> Product1/2
  theta/1 -> Sum2/2
  phi/1 -> Sum5/2
  Sum2/1 -> [theta_err]
  X0_desired2/1 -> phi-launch/1, "theta-launch "/1
  "theta-launch "/1 -> Sum2/1
  [phi_err] -> Product3/2
  [theta_err] -> Product2/2
  Sum5/1 -> [phi_err]
  phi-launch/1 -> Sum5/1

== system flatball_6dof_candp_wrk/flatball-6dof-CandP/aero-coefficients/Subsystem ==
  alpha3 : Inport
  1-D Lookup Table : Lookup_n-D  NumberOfTableDimensions=1  BreakpointsForDimension1=disc.aoa_data  Table=disc.Cdrag_data  InterpMethod=Cubic spline  ExtrapMethod=Cubic spline  InternalRulePriority=Speed  RndMeth=Simplest  InputSameDT=on
  Math Function : Math  Operator=square  SaturateOnIntegerOverflow=on
  Product1 : Product  Inputs=**
  Sum1 : Sum
  Sum2 : Sum  Inputs=+-
  Terminator : Terminator
  mg : Constant  Value=disc.CD0
  mg1 : Constant  Value=disc.CDa
  mg2 : Constant  Value=disc.alpha0
  Cdrag : Outport
  wires:
  alpha3/1 -> 1-D Lookup Table/1, Sum2/1
  mg1/1 -> Product1/1
  mg/1 -> Sum1/1
  Product1/1 -> Sum1/2
  Sum2/1 -> Math Function/1
  mg2/1 -> Sum2/2
  Math Function/1 -> Product1/2
  1-D Lookup Table/1 -> Cdrag/1
  Sum1/1 -> Terminator/1

== system flatball_6dof_candp_wrk/flatball-6dof-CandP/aero-coefficients/Subsystem1 ==
  alpha3 : Inport
  1-D Lookup Table : Lookup_n-D  NumberOfTableDimensions=1  BreakpointsForDimension1=disc.aoa_data  Table=disc.Clift_data  InterpMethod=Cubic spline  ExtrapMethod=Cubic spline  InternalRulePriority=Speed  RndMeth=Simplest  InputSameDT=on
  Product1 : Product  Inputs=**
  Sum1 : Sum
  Terminator : Terminator
  mg : Constant  Value=disc.CL0
  mg1 : Constant  Value=disc.CLa
  Clift : Outport
  wires:
  Product1/1 -> Sum1/2
  mg/1 -> Sum1/1
  mg1/1 -> Product1/1
  alpha3/1 -> 1-D Lookup Table/1, Product1/2
  1-D Lookup Table/1 -> Clift/1
  Sum1/1 -> Terminator/1

== system flatball_6dof_candp_wrk/flatball-6dof-CandP/aero-coefficients/Subsystem2 ==
  dTH3dt : Inport
  alpha3 : Inport  Port=2
  v_inf : Inport  Port=3
  1-D Lookup Table : Lookup_n-D  NumberOfTableDimensions=1  BreakpointsForDimension1=disc.aoa_data  Table=disc.CM_data  InterpMethod=Cubic spline  ExtrapMethod=Cubic spline  InternalRulePriority=Speed  RndMeth=Simplest  InputSameDT=on
  Gain : Gain  Gain=2
  Product1 : Product  Inputs=**
  Product2 : Product  Inputs=*/
  Product3 : Product  Inputs=**
  Product4 : Product  Inputs=**
  Selector : Selector  InputPortWidth=3  IndexOptions=Index vector (dialog)  Indices=[2]  OutputSizes=1
  Sum1 : Sum
  Sum2 : Sum
  Terminator : Terminator
  mg : Constant  Value=disc.CM0
  mg1 : Constant  Value=disc.CMa
  mg2 : Constant  Value=disc.c
  mg3 : Constant  Value=disc.CMq
  CM : Outport
  wires:
  mg2/1 -> Product2/1
  Gain/1 -> Product2/2
  v_inf/1 -> Gain/1
  mg1/1 -> Product1/2
  alpha3/1 -> 1-D Lookup Table/1, Product1/1
  dTH3dt/1 -> Selector/1
  Product2/1 -> Product3/2
  Product3/1 -> Product4/2
  mg3/1 -> Product4/1
  Selector/1 -> Product3/1  "q3"
  Product1/1 -> Sum2/2
  1-D Lookup Table/1 -> Sum1/1
  mg/1 -> Sum2/1
  Sum2/1 -> Terminator/1
  Product4/1 -> Sum1/2
  Sum1/1 -> CM/1

== system flatball_6dof_candp_wrk/flatball-6dof-CandP/aero-coefficients/Subsystem3 ==
  dTH3dt : Inport
  v_inf : Inport  Port=2
  Gain : Gain  Gain=2
  Product1 : Product  Inputs=**
  Product2 : Product  Inputs=*/
  Product3 : Product  Inputs=**
  Selector : Selector  InputPortWidth=3  IndexOptions=Index vector (dialog)  Indices=[1]  OutputSizes=1
  mg1 : Constant  Value=disc.CLp
  mg2 : Constant  Value=disc.c
  CL : Outport
  wires:
  Product3/1 -> CL/1
  mg1/1 -> Product1/1
  v_inf/1 -> Gain/1
  mg2/1 -> Product2/1
  dTH3dt/1 -> Selector/1
  Product1/1 -> Product3/1
  Product2/1 -> Product3/2
  Gain/1 -> Product2/2
  Selector/1 -> Product1/2  "p3"

== system flatball_6dof_candp_wrk/flatball-6dof-CandP/aero-coefficients/Subsystem4 ==
  dTH3dt : Inport
  v_inf : Inport  Port=2
  Gain : Gain  Gain=2
  Product2 : Product  Inputs=*/
  Product3 : Product  Inputs=**
  Product4 : Product  Inputs=**
  Selector : Selector  InputPortWidth=3  IndexOptions=Index vector (dialog)  Indices=[3]  OutputSizes=1
  mg2 : Constant  Value=disc.c
  mg3 : Constant  Value=disc.CNr
  CN : Outport
  wires:
  mg3/1 -> Product4/1
  Product3/1 -> Product4/2
  Product2/1 -> Product3/2
  dTH3dt/1 -> Selector/1
  v_inf/1 -> Gain/1
  Gain/1 -> Product2/2
  mg2/1 -> Product2/1
  Product4/1 -> CN/1
  Selector/1 -> Product3/1  "r3"

== system flatball_6dof_candp_wrk/flatball-6dof-CandP/aero-coefficients/Subsystem5 ==
  dTH3dt : Inport
  v_inf : Inport  Port=2
  Ground : Ground
  Terminator : Terminator
  Terminator1 : Terminator
  Cside : Outport
  wires:
  dTH3dt/1 -> Terminator/1
  Ground/1 -> Cside/1
  v_inf/1 -> Terminator1/1

== system flatball_6dof_candp_wrk/flatball-6dof-CandP/aero-coefficients/alpha3 ==
  dX3dt : Inport
  Atan2 : Trigonometry  Operator=atan2
  Selector : Selector  InputPortWidth=3  IndexOptions=Index vector (dialog)  Indices=[3]  OutputSizes=1
  Selector3 : Selector  InputPortWidth=3  IndexOptions=Index vector (dialog)  Indices=[1]  OutputSizes=1
  alpha3 : Outport
  tag scope: alpha3=scoped
  wires:
  dX3dt/1 -> Selector/1, Selector3/1
  Selector3/1 -> Atan2/2  "u3"
  Selector/1 -> Atan2/1  "w3"
  Atan2/1 -> alpha3/1, [alpha3]  "alpha"

== system flatball_6dof_candp_wrk/flatball-6dof-CandP/earth-reference/v_inf ==
  dX2dt : Inport
  Sqrt : Sqrt  SaturateOnIntegerOverflow=on
  Square3 : Math  Operator=square  SaturateOnIntegerOverflow=on
  Sum1 : Sum  Inputs=1
  tag scope: v_inf=scoped
  wires:
  Sqrt/1 -> [v_inf]  "v_inf"
  dX2dt/1 -> Square3/1
  Square3/1 -> Sum1/1
  Sum1/1 -> Sqrt/1

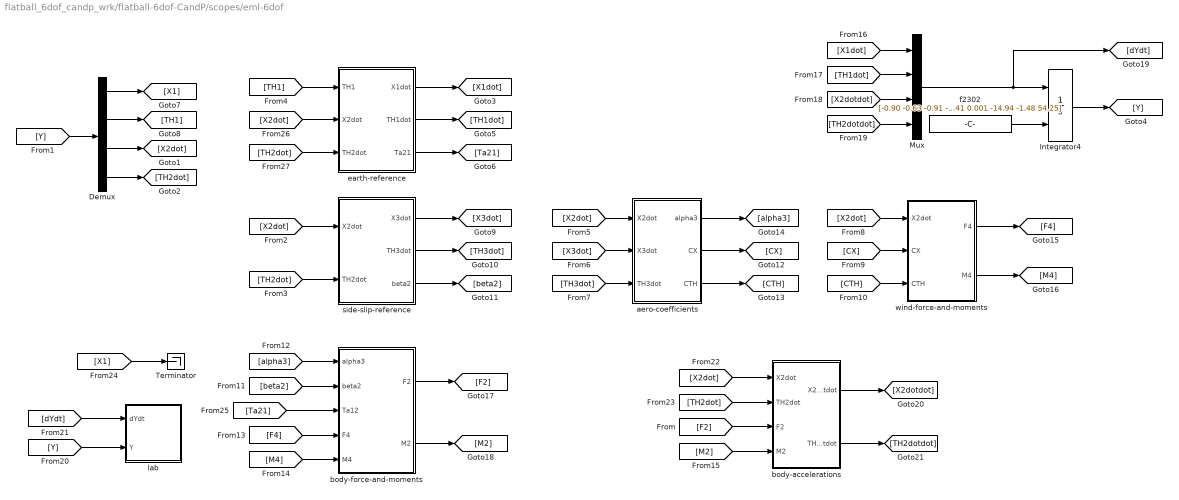
== system flatball_6dof_candp_wrk/flatball-6dof-CandP/scopes/eml-6dof ==
  Demux : Demux  Outputs=[3 3 3 3]
  Integrator4 : Integrator  InitialConditionSource=external
  Mux : Mux
  Terminator : Terminator
  aero-coefficients : MATLAB Function  TreatAsAtomicUnit=on
  body-accelerations : MATLAB Function  TreatAsAtomicUnit=on
  body-force-and-moments : MATLAB Function  TreatAsAtomicUnit=on
  earth-reference : MATLAB Function  TreatAsAtomicUnit=on
  f2302 : Constant  Value=[-0.90 -0.63 -0.91 -0.07 0.21 5.03 13.42 -0.41 0.001 -14.94 -1.48 54.25]
  lab : Subsystem
  side-slip-reference : MATLAB Function  TreatAsAtomicUnit=on
  wind-force-and-moments : MATLAB Function  TreatAsAtomicUnit=on
  wires:
  earth-reference/1(X1dot) -> [X1dot]
  earth-reference/2(TH1dot) -> [TH1dot]
  earth-reference/3(Ta21) -> [Ta21]
  [Y] -> Demux/1
  Demux/1 -> [X1]
  Demux/2 -> [TH1]
  Demux/3 -> [X2dot]
  Demux/4 -> [TH2dot]
  [X2dot] -> side-slip-reference/1(X2dot)
  [TH2dot] -> side-slip-reference/2(TH2dot)
  side-slip-reference/1(X3dot) -> [X3dot]
  side-slip-reference/2(TH3dot) -> [TH3dot]
  side-slip-reference/3(beta2) -> [beta2]
  [TH1] -> earth-reference/1(TH1)
  [X2dot] -> aero-coefficients/1(X2dot)
  [X3dot] -> aero-coefficients/2(X3dot)
  [TH3dot] -> aero-coefficients/3(TH3dot)
  aero-coefficients/3(CTH) -> [CTH]
  aero-coefficients/2(CX) -> [CX]
  aero-coefficients/1(alpha3) -> [alpha3]
  [X2dot] -> wind-force-and-moments/1(X2dot)
  [CX] -> wind-force-and-moments/2(CX)
  [CTH] -> wind-force-and-moments/3(CTH)
  [beta2] -> body-force-and-moments/2(beta2)
  [alpha3] -> body-force-and-moments/1(alpha3)
  wind-force-and-moments/1(F4) -> [F4]
  wind-force-and-moments/2(M4) -> [M4]
  [F4] -> body-force-and-moments/4(F4)
  [M4] -> body-force-and-moments/5(M4)
  body-force-and-moments/1(F2) -> [F2]
  body-force-and-moments/2(M2) -> [M2]
  [TH2dotdot] -> Mux/4
  Mux/1 -> Integrator4/1, [dYdt]
  [TH1dot] -> Mux/2
  [X1dot] -> Mux/1
  f2302/1 -> Integrator4/2
  [X2dotdot] -> Mux/3
  Integrator4/1 -> [Y]
  [dYdt] -> lab/1(dYdt)
  [Y] -> lab/2(Y)
  [F2] -> body-accelerations/3(F2)
  [M2] -> body-accelerations/4(M2)
  [X2dot] -> body-accelerations/1(X2dot)
  [TH2dot] -> body-accelerations/2(TH2dot)
  body-accelerations/2(TH2dotdot) -> [TH2dotdot]
  body-accelerations/1(X2dotdot) -> [X2dotdot]
  [Ta21] -> body-force-and-moments/3(Ta12)
  [X1] -> Terminator/1
  [X2dot] -> earth-reference/2(X2dot)
  [TH2dot] -> earth-reference/3(TH2dot)

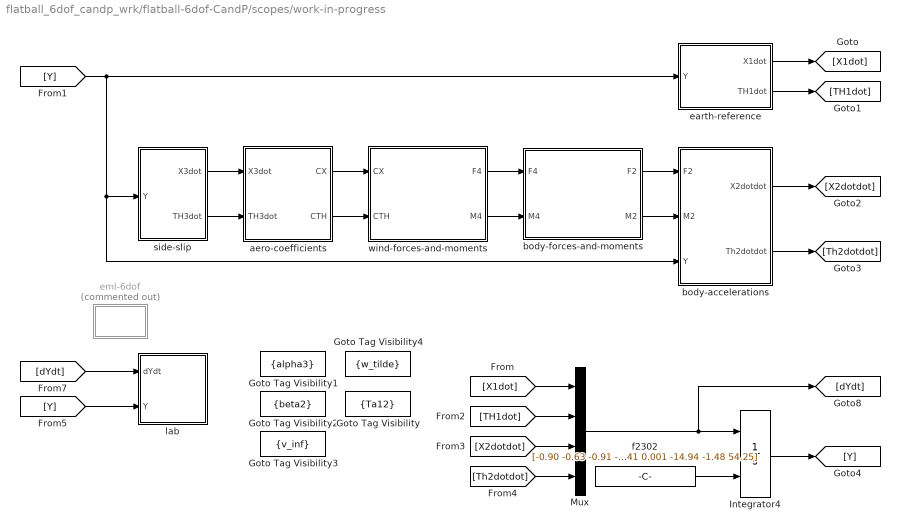
== system flatball_6dof_candp_wrk/flatball-6dof-CandP/scopes/work-in-progress ==
  Goto Tag Visibility : GotoTagVisibility  GotoTag=Ta12
  Goto Tag Visibility1 : GotoTagVisibility  GotoTag=alpha3
  Goto Tag Visibility2 : GotoTagVisibility  GotoTag=beta2
  Goto Tag Visibility3 : GotoTagVisibility  GotoTag=v_inf
  Goto Tag Visibility4 : GotoTagVisibility  GotoTag=w_tilde
  Integrator4 : Integrator  InitialConditionSource=external
  Mux : Mux
  aero-coefficients : Subsystem
  body-accelerations : Subsystem
  body-forces-and-moments : Subsystem
  earth-reference : Subsystem
  eml-6dof : Subsystem  Commented=on
  f2302 : Constant  Value=[-0.90 -0.63 -0.91 -0.07 0.21 5.03 13.42 -0.41 0.001 -14.94 -1.48 54.25]
  lab : Subsystem
  side-slip : Subsystem
  wind-forces-and-moments : Subsystem
  wires:
  [X1dot] -> Mux/1
  [Y] -> lab/2(Y)
  [X2dotdot] -> Mux/3
  [Th2dotdot] -> Mux/4
  [dYdt] -> lab/1(dYdt)
  [TH1dot] -> Mux/2
  body-accelerations/1(X2dotdot) -> [X2dotdot]
  Mux/1 -> [dYdt], Integrator4/1
  Integrator4/1 -> [Y]
  [Y] -> earth-reference/1(Y), side-slip/1(Y), body-accelerations/3(Y)
  f2302/1 -> Integrator4/2
  body-accelerations/2(Th2dotdot) -> [Th2dotdot]
  earth-reference/2(TH1dot) -> [TH1dot]
  earth-reference/1(X1dot) -> [X1dot]
  body-forces-and-moments/2(M2) -> body-accelerations/2(M2)
  wind-forces-and-moments/2(M4) -> body-forces-and-moments/2(M4)
  wind-forces-and-moments/1(F4) -> body-forces-and-moments/1(F4)
  side-slip/2(TH3dot) -> aero-coefficients/2(TH3dot)
  body-forces-and-moments/1(F2) -> body-accelerations/1(F2)
  aero-coefficients/1(CX) -> wind-forces-and-moments/1(CX)
  side-slip/1(X3dot) -> aero-coefficients/1(X3dot)
  aero-coefficients/2(CTH) -> wind-forces-and-moments/2(CTH)

== system flatball_6dof_candp_wrk/flatball-6dof-CandP/wind-forces-and-moments/Subsystem ==
  v_inf : Inport
  Gain2 : Gain  Gain=0.5
  Math Function : Math  Operator=square  SaturateOnIntegerOverflow=on
  Product : Product
  Product1 : Product
  Product2 : Product
  S : Constant  Value=disc.S
  c : Constant  Value=disc.c
  rho : Constant  Value=amb.rho
  qS : Outport
  qSc : Outport  Port=2
  wires:
  rho/1 -> Gain2/1
  Gain2/1 -> Product/2
  Math Function/1 -> Product/1
  v_inf/1 -> Math Function/1
  Product/1 -> Product1/1  "q_inf"
  Product1/1 -> Product2/1, qS/1
  Product2/1 -> qSc/1
  c/1 -> Product2/2
  S/1 -> Product1/2

== system flatball_6dof_candp_wrk/flatball-6dof-CandP/zero-side-slip-reference/beta2 ==
  dX2dt : Inport
  Atan2 : Trigonometry  Operator=atan2
  Goto3 : Goto  Commented=on  GotoTag=beta2  TagVisibility=scoped
  Selector : Selector  InputPortWidth=3  IndexOptions=Index vector (dialog)  Indices=[2]  OutputSizes=1
  Selector3 : Selector  InputPortWidth=3  IndexOptions=Index vector (dialog)  Indices=[1]  OutputSizes=1
  beta2 : Outport
  wires:
  dX2dt/1 -> Selector/1, Selector3/1
  Selector3/1 -> Atan2/2  "u2"
  Selector/1 -> Atan2/1  "v2"
  Atan2/1 -> beta2/1, Goto3/1  "beta"
